simulink model "PV_MPPT_DesktopSim"  (R2023b)
settings: Solver=ode23tb  StartTime=0.0  StopTime=inf  MaxStep=1e-4  RelTol=1e-3
PreLoadFcn:
  | load('EmulatedPV_LowPowerData.mat');
  | 
  | numIrr = 10;
  | ArrayPower = ArrayCurrent.*ArrayVoltage;
InitFcn:
  | Ts = 1e-4;
  | Tc = Ts;
undefined symbols (not defined in the file): ArrayCurrent, ArrayVoltage, DiscIntNeverNeededParam, Irradiance, Tdata
libraries: spsSeriesRLCBranchLib x27, fl_lib x15, spsMosfetLib x11, ee_lib x11, spsVoltageMeasurementLib x7, spsCurrentMeasurementLib x6, nesl_utility x5, spsDiodeLib x5, spspowerguiLib x4, spsTriangleGeneratorLib x3, spsParallelRLCBranchLib x3, spsGroundLib x2
(part 1 of 3)
settings Model: Creator=mmishra  LastModifiedBy=32295
settings SolverCC: AlgebraicLoopSolver=TrustRegion
settings DataIOCC: ReturnWorkspaceOutputs=off
settings DebuggingCC: UnconnectedInputMsg=warning  UnconnectedOutputMsg=warning  UnconnectedLineMsg=warning  ArithmeticOperatorsInVariantConditions=warning
settings ModelReferenceCC: EnableRefExpFcnMdlSchedulingChecks=on
settings SFSimCC: SimUseLocalCustomCode=off  CustomCodeUndefinedFunction=UseInterfaceOnly
settings RTWCC: RTWUseLocalCustomCode=off

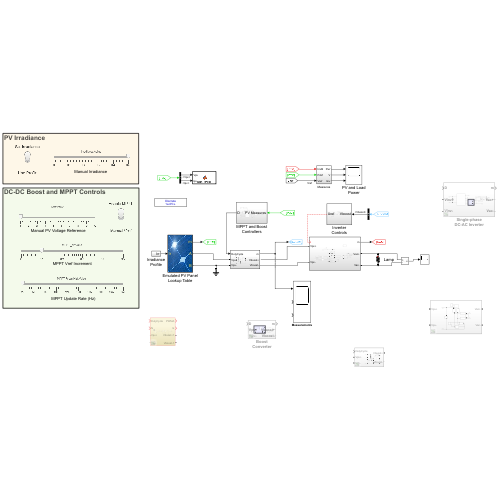
[thumbnail: Simulink's stored preview of the top-level diagram]
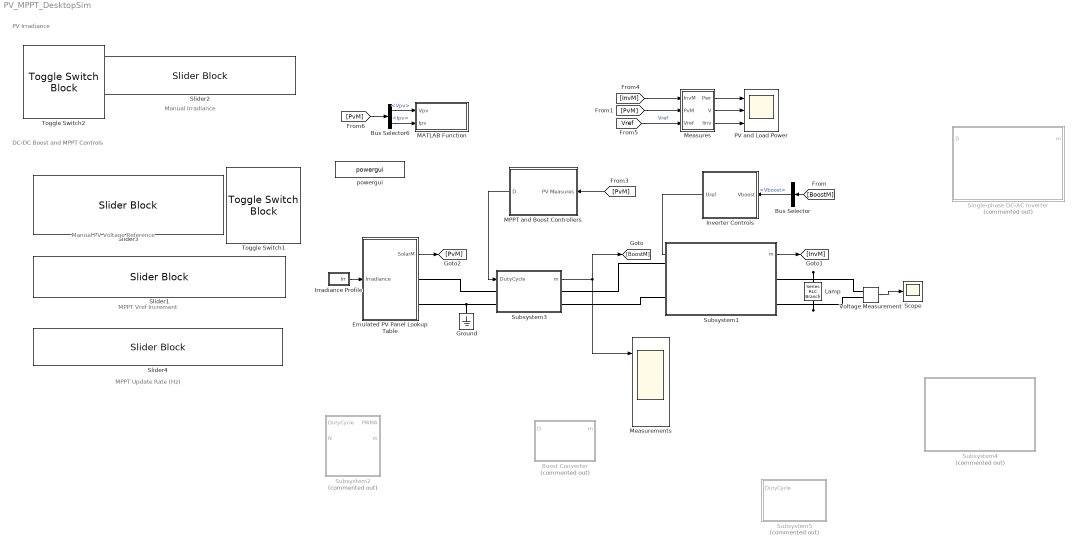
== system PV_MPPT_DesktopSim ==
  note: Manual Irradiance
  note: PV Irradiance
  note: MPPT Update Rate (Hz)
  note: MPPT Vref Increment
  note: DC-DC Boost and MPPT Controls
  note: Manual PV Voltage Reference
  Boost Converter : Subsystem  Commented=on
  Bus Selector : BusSelector  OutputSignals=Vboost
  Bus Selector6 : BusSelector  OutputSignals=Vpv,Ipv
  Emulated PV Panel Lookup Table : Subsystem
      mask Display:
      | image(imread('panel.jpg'))
      | color('yellow')
      | port_label('input',1,'Ir')
      | port_label('output',1,'m')
      | port_label('Rconn',1,'A')
      | port_label('Rconn',2,'B')
  Ground : spsGroundLib/Ground  LConnTagsString=a
  Inverter Controls : Subsystem
  Irradiance Profile : Subsystem
  Lamp : spsSeriesRLCBranchLib/Series RLC Branch  LConnTagsString=__new0  RConnTagsString=__new0  BranchType=R  Resistance=11.5  Inductance=1e-3  SetiL0=off  InitialCurrent=0  Capacitance=1e-6  Setx0=off  InitialVoltage=0  Measurements=None
  MATLAB Function : MATLAB Function  TreatAsAtomicUnit=on  SystemSampleTime=1/20
  MPPT and Boost Controllers : Subsystem
  Measurements : Scope  NumInputPorts=3
  Measures : Subsystem
  PV and Load Power : Scope  NumInputPorts=3
  Scope : Scope
  Single-phase DC-AC Inverter : Subsystem  Commented=on
  Slider1 : SliderBlock  ScaleMax=0.5  TickInterval=0.10000000000000001
  Slider2 : SliderBlock  ScaleMax=0.5  TickInterval=0.10000000000000001
  Slider3 : SliderBlock  ScaleMin=1  ScaleMax=10  TickInterval=1
  Slider4 : SliderBlock  ScaleMin=25  ScaleMax=250  TickInterval=25
  Subsystem1 : Subsystem
  Subsystem2 : Subsystem  Commented=on
  Subsystem3 : Subsystem
  Subsystem4 : Subsystem  Commented=on
  Subsystem5 : Subsystem  Commented=on
  Toggle Switch1 : ToggleSwitchBlock  LabelPosition=Hide
      settings: Values={{'Manual Vref', 'Enable MPPT'}, [0 1]}
  Toggle Switch2 : ToggleSwitchBlock  LabelPosition=Hide
      settings: Values={{'Use Profile', 'Set Irradiance'}, [0 1]}
  Voltage Measurement : spsVoltageMeasurementLib/Voltage Measurement  PhasorSimulation=off  OutputType=Complex  PSBequivalent=0
  powergui : spspowerguiLib/powergui  Priority=1  SimulationMode=Discrete  SampleTime=1e-5  frequency=60  Iterations=50  frequencyindice=0  Pbase=100e6  ErrMax=1e-4  UnitsV=kV  UnitsW=MW  buscounter=0  FunctionMessages=off  echomessages=off  EnableUseOfTLC=off  CurrentSourceSwitches=off  DisableSnubberDevices=off  DisableRonSwitches=off  DisableVfSwitches=off  DisplayEquations=off  AutomaticDiscreteSolvers=off  SolverType=Tustin  Interpol=off  ExternalGateDelay=off  methode=off  Ts=0  x0status=blocks  SPID=off  SwTol=0  HookPort=off  NonlinearTolerance=1e-4  nMaxIteration=100  ContinueOnMaxIteration=off  RestoreLinks=warning  ResistiveCurrentMeasurement=off  Frange=[0:2:500]  Ylog=off  Xlog=on  ShowGrid=off  save=off  variable=ZData  structure=0  ZoomFFT=on  StartTime=0.0  cycles=1  DisplayStyle=1  fundamental=60  FreqAxis=off  MaxFrequency=1000  frequencyindicesteady=1  RmsSteady=1  display=off
  wires:
  Irradiance Profile/1(Irr) -> Emulated PV Panel Lookup Table/1(Irradiance)
  Subsystem1/1(m) -> [InvM]
  Emulated PV Panel Lookup Table/1(SolarM) -> [PvM]
  MPPT and Boost Controllers/1(D) -> Subsystem3/1(DutyCycle)
  Subsystem3/1(m) -> Measurements/1, [BoostM]
  [PvM] -> MPPT and Boost Controllers/1(PV Measures)
  Bus Selector/1 -> Inverter Controls/1(Vboost)  "<Vboost>"
  Inverter Controls/1(Uref) -> ?
  [BoostM] -> Bus Selector/1
  Bus Selector6/1 -> MATLAB Function/1(Vpv)  "<Vpv>"
  Bus Selector6/2 -> MATLAB Function/2(Ipv)  "<Ipv>"
  [PvM] -> Bus Selector6/1
  [InvM] -> Measures/1(InvM)
  [PvM] -> Measures/2(PvM)
  [Vref] -> Measures/3(Vref)  "Vref"
  Measures/1(Pwr) -> PV and Load Power/1
  Measures/2(V) -> PV and Load Power/2
  Measures/3(Iinv) -> PV and Load Power/3
  Voltage Measurement/1 -> Scope/1
  connections:
  Ground/LConn1 -- Subsystem3/LConn2 -- Emulated PV Panel Lookup Table/RConn2
  Subsystem3/LConn1 -- Emulated PV Panel Lookup Table/RConn1
  Lamp/RConn1 -- Subsystem1/RConn2 -- Voltage Measurement/LConn2
  Subsystem3/RConn1 -- Subsystem1/LConn1
  Subsystem3/RConn2 -- Subsystem1/LConn2
  Lamp/LConn1 -- Subsystem1/RConn1 -- Voltage Measurement/LConn1

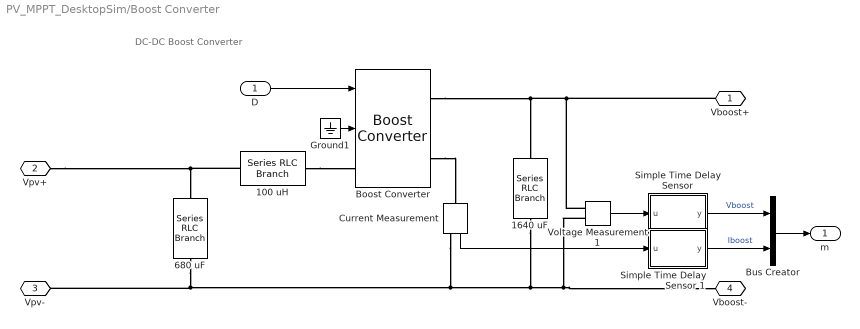
== system PV_MPPT_DesktopSim/Boost Converter ==
  note: DC-DC Boost Converter
  D : Inport
  100 uH : spsSeriesRLCBranchLib/Series RLC Branch  LConnTagsString=__new0  RConnTagsString=__new0  BranchType=L  Resistance=1  Inductance=100e-6  SetiL0=off  InitialCurrent=0  Capacitance=1e-6  Setx0=off  InitialVoltage=0  Measurements=None
  1640 uF : spsSeriesRLCBranchLib/Series RLC Branch  LConnTagsString=__new0  RConnTagsString=__new0  BranchType=C  Resistance=1  Inductance=1e-3  SetiL0=off  InitialCurrent=0  Capacitance=1640e-6  Setx0=off  InitialVoltage=30  Measurements=None
  680 uF : spsSeriesRLCBranchLib/Series RLC Branch  LConnTagsString=__new0  RConnTagsString=__new0  BranchType=C  Resistance=1e-3  Inductance=1e-3  SetiL0=off  InitialCurrent=0  Capacitance=680e-6  Setx0=off  InitialVoltage=20  Measurements=None
  "Boost Converter " : spsBoostConverterLib/Boost Converter  ModelType=Average model (D-controlled)  Ron=1e-3  Rs=1e6  Cs=inf  Vforward=[0,0.8]  Ron_Diode=1e-3  Rs_Diode=1e6  Cs_Diode=inf  Vf_Diode=0.8  Rs_CurrentSource=inf  Ron_ACsource=1e-3
      settings: LibrarySourceBlock=sps_lib/Power Electronics/Boost Converter
  Bus Creator : BusCreator  Inputs=2
  Current Measurement : spsCurrentMeasurementLib/Current Measurement  PhasorSimulation=off  OutputType=Complex  PSBequivalent=0
  Ground1 : Ground
  "Simple Time Delay Sensor " : Subsystem  mask{Ts=Ts, Tau=0.0001}
      mask prompts: Ts "Sample Time, [s]"; Tau "Time Constant, Tau [s]"
      mask help: Simple Sensor
      mask Display: fprintf('1\n------------\n(1 + s Tau)');
  Simple Time Delay Sensor 1 : Subsystem  mask{Ts=Ts, Tau=0.0001}
      mask prompts: Ts "Sample Time, [s]"; Tau "Time Constant, Tau [s]"
      mask help: Simple Sensor
      mask Display: fprintf('1\n------------\n(1 + s Tau)');
  Voltage Measurement1 : spsVoltageMeasurementLib/Voltage Measurement  PhasorSimulation=off  OutputType=Complex  PSBequivalent=0
  Vboost+ : PMIOPort  Side=Right
  Vpv+ : PMIOPort  Port=2  Side=Left
  Vpv- : PMIOPort  Port=3  Side=Left
  Vboost- : PMIOPort  Port=4  Side=Right
  m : Outport  VectorParamsAs1DForOutWhenUnconnected=off
  wires:
  Ground1/1 -> "Boost Converter "/2
  Current Measurement/1 -> Simple Time Delay Sensor 1/1(u)
  Voltage Measurement1/1 -> "Simple Time Delay Sensor "/1(u)
  Bus Creator/1 -> m/1
  "Simple Time Delay Sensor "/1(y) -> Bus Creator/1  "Vboost"
  Simple Time Delay Sensor 1/1(y) -> Bus Creator/2  "Iboost"
  D/1 -> "Boost Converter "/1
  connections:
  100 uH/LConn1 -- Vpv+/RConn1 -- 680 uF/LConn1
  "Boost Converter "/RConn2 -- Current Measurement/LConn1
  100 uH/RConn1 -- "Boost Converter "/LConn1
  Voltage Measurement1/LConn1 -- Vboost+/RConn1 -- "Boost Converter "/RConn1 -- 1640 uF/LConn1
  680 uF/RConn1 -- Vboost-/RConn1 -- Voltage Measurement1/LConn2 -- 1640 uF/RConn1 -- Current Measurement/RConn1 -- Vpv-/RConn1

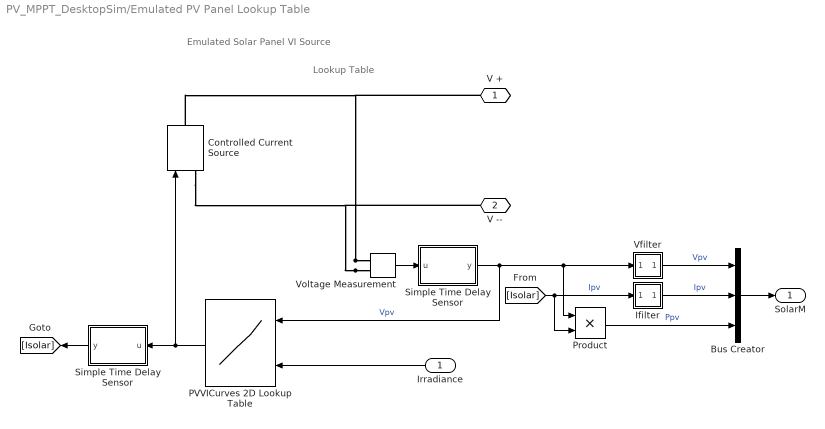
== system PV_MPPT_DesktopSim/Emulated PV Panel Lookup Table ==
  note: Lookup Table
  note: Emulated Solar Panel VI Source
  Irradiance : Inport
  Bus Creator : BusCreator  Inputs=3
  Controlled Current Source : spsControlledCurrentSourceLib/Controlled Current Source  Initialize=on  Source_Type=AC  Amplitude=0  Phase=0  Frequency=0  Measurements=None
  Ifilter : Subsystem  mask{Tf=0.01}
      mask prompts: Tf "Filter Time Constant"
  PVVICurves 2D Lookup Table : Lookup_n-D  BreakpointsForDimension1=ArrayVoltage  BreakpointsForDimension2=Irradiance  Table=ArrayCurrent  InternalRulePriority=Speed  RndMeth=Simplest
      settings: InputPortMap=u0,u1
  Product : Product
  Simple Time Delay Sensor : Subsystem  mask{Ts=Ts, Tau=0.0001}
      mask prompts: Ts "Sample Time, [s]"; Tau "Time Constant, Tau [s]"
      mask help: Simple Sensor
      mask Display: fprintf('1\n------------\n(1 + s Tau)');
  "Simple Time Delay Sensor " : Subsystem  mask{Ts=Ts, Tau=0.0001}
      mask prompts: Ts "Sample Time, [s]"; Tau "Time Constant, Tau [s]"
      mask help: Simple Sensor
      mask Display: fprintf('1\n------------\n(1 + s Tau)');
  Vfilter : Subsystem  mask{Tf=0.01}
      mask prompts: Tf "Filter Time Constant"
  Voltage Measurement : spsVoltageMeasurementLib/Voltage Measurement  PhasorSimulation=off  OutputType=Complex  PSBequivalent=0
  V + : PMIOPort  Side=Right
  V -- : PMIOPort  Port=2  Side=Right
  SolarM : Outport  VectorParamsAs1DForOutWhenUnconnected=off
  wires:
  Irradiance/1 -> PVVICurves 2D Lookup Table/2
  PVVICurves 2D Lookup Table/1 -> Simple Time Delay Sensor/1(u), Controlled Current Source/1
  Bus Creator/1 -> SolarM/1
  [Isolar] -> Product/2, Ifilter/1(u)  "Ipv"
  Product/1 -> Bus Creator/3  "Ppv"
  Simple Time Delay Sensor/1(y) -> [Isolar]
  "Simple Time Delay Sensor "/1(y) -> Product/1, Vfilter/1(u), PVVICurves 2D Lookup Table/1  "Vpv"
  Voltage Measurement/1 -> "Simple Time Delay Sensor "/1(u)
  Vfilter/1(y) -> Bus Creator/1  "Vpv"
  Ifilter/1(y) -> Bus Creator/2  "Ipv"
  connections:
  Voltage Measurement/LConn2 -- Controlled Current Source/LConn1 -- V --/RConn1
  Voltage Measurement/LConn1 -- Controlled Current Source/RConn1 -- V +/RConn1

== system PV_MPPT_DesktopSim/Inverter Controls ==
  Vboost : Inport
  Boost Voltage Controller : slpidlib/PID Controller  Controller=PI  Form=Parallel  TimeDomain=Discrete-time  UseExternalTs=off  SampleTime=Tc  IntegratorMethod=Forward Euler  FilterMethod=Forward Euler  ControllerParametersSource=internal  P=3  I=250  UseKiTs=off  D=0  N=100  UseFilter=on  TunerSelectOption=Transfer Function Based (PID Tuner App)  InitialConditionSource=internal  InitialConditionForIntegrator=1  InitialConditionForFilter=0  DifferentiatorICPrevScaledInput=0  ExternalReset=none  TrackingMode=off  Kt=1  LimitOutput=on  SatLimitsSource=internal  UpperSaturationLimit=1  LowerSaturationLimit=0  LinearizeAsGain=on  AntiWindupMode=clamping  Kb=1  LimitIntegrator=off  UpperIntegratorSaturationLimit=inf  LowerIntegratorSaturationLimit=-inf  POutMin=[]  POutMax=[]  IOutMin=[]  IOutMax=[]  DOutMin=[]  DOutMax=[]  NOutMin=[]  NOutMax=[]  SumOutMin=[]  SumOutMax=[]  SaturationOutMin=[]  SaturationOutMax=[]  PParamMin=[]  PParamMax=[]  IParamMin=[]  IParamMax=[]  DParamMin=[]  DParamMax=[]  NParamMin=[]  NParamMax=[]  KbParamMin=[]  KbParamMax=[]  KtParamMin=[]  KtParamMax=[]  KbOutMin=[]  KbOutMax=[]  KtOutMin=[]  KtOutMax=[]  IntegratorOutMin=[]  IntegratorOutMax=[]  FilterOutMin=[]  FilterOutMax=[]  SumI1OutMin=[]  SumI1OutMax=[]  SumI2OutMin=[]  SumI2OutMax=[]  SumI3OutMin=[]  SumI3OutMax=[]  SumI4OutMin=[]  SumI4OutMax=[]  SumDOutMin=[]  SumDOutMax=[]  DifferentiatorOutMin=[]  DifferentiatorOutMax=[]  FilterDiffOutCoefMin=[]  FilterDiffOutCoefMax=[]  ReciprocalOutMin=[]  ReciprocalOutMax=[]  SumDenOutMin=[]  SumDenOutMax=[]  SumNumOutMin=[]  SumNumOutMax=[]  DivideOutMin=[]  DivideOutMax=[]  UdiffTsProdOutMin=[]  UdiffTsProdOutMax=[]  NTsProdOutMin=[]  NTsProdOutMax=[]  UintegralTsProdOutMin=[]  UintegralTsProdOutMax=[]  UngainTsProdOutMin=[]  UngainTsProdOutMax=[]  ClampingZeroOutDataTypeStr=Inherit: Inherit via back propagation  ClampingZeroOutMin=[]  ClampingZeroOutMax=[]  FilterDenConstantOutDataTypeStr=Inherit: Inherit via back propagation  FilterDenConstantOutMin=[]  FilterDenConstantOutMax=[]  PCopyOutDataTypeStr=Inherit: Inherit via back propagation  PCopyOutMin=[]  PCopyOutMax=[]  NCopyOutDataTypeStr=Inherit: Inherit via back propagation  NCopyOutMin=[]  NCopyOutMax=[]  IntegratorContinuousStateAttributes=''  IntegratorStateMustResolveToSignalObject=off  IntegratorRTWStateStorageClass=Auto  FilterContinuousStateAttributes=''  FilterStateMustResolveToSignalObject=off  FilterRTWStateStorageClass=Auto  ParallelPVariant=InternalParameters  IdealPVariant=Disabled  IVariant=InternalParameters  DVariant=Disabled  IntegratorVariant=Discrete  SatVariant=Enabled  AWVariant=DiscClampingParallel  PCopyVariant=Disabled  TRVariant=Disabled  FdbkBlocksVariant=Forward  IdealPFdbkVariant=Disabled  SatFdbkVariant=Disabled  DerivativeFilterVariant=Disabled  NVariant=Disabled  NCopyVariant=Disabled_SignalSpec  FilterICVariant=Disabled  IntegratorICVariant=InternalICs  ExternalResetVariant=Disabled  TRSumVariant=Passthrough  SumFdbkVariant=Disabled  SumVariant=Sum_PI  TsampFilterVariant=InternalTs  TsampNgainVariant=Passthrough  TsampIntegralVariant=Disabled_SignalSpec  ExternalSaturationOutDataTypeStr=Inherit: Same as second input
  Constant1 : Constant  Value=30
  Gain : Gain  Gain=1/30
  "PWM Generator (2-Level) " : spsPWMGenerator2LevelLib/PWM Generator (2-Level)  Commented=through  ModulatorType=Single-phase full-bridge (4 pulses)  ModulatorMode=Unsynchronized  Fc=6000  Pc=90  nF=27  MinMax="[ -1  1 ]"  SamplingTechnique=Natural  ModulatingSignals=off  m=0.8  Freq=60  Phase=0  Ts=Ts  ShowCarrierOutport=off
  Product : Product
  Sine Wave : Sin  Frequency=2*pi*60  SampleTime=Tc
  Sum3 : Sum  Inputs=|+-
  Uref : Outport  VectorParamsAs1DForOutWhenUnconnected=off
  wires:
  Constant1/1 -> Sum3/2
  Sine Wave/1 -> Product/1
  Boost Voltage Controller/1 -> Product/2
  Sum3/1 -> Gain/1
  Vboost/1 -> Sum3/1
  Gain/1 -> Boost Voltage Controller/1
  Product/1 -> "PWM Generator (2-Level) "/1
  "PWM Generator (2-Level) "/1 -> Uref/1

== system PV_MPPT_DesktopSim/Irradiance Profile ==
  note: PV Irradiance
  Irradiance : Constant  Value=0.5  OutDataTypeStr=single
  Irradiance_Select : Constant  OutDataTypeStr=single
  NewIrradiance1 : Constant  Value=0.15  OutDataTypeStr=single
  Pulse Generator : DiscretePulseGenerator  PulseType=Time based  Amplitude=0.15  Period=10  PulseWidth=50
  Sum : Sum  Inputs=|++
  Switch : Switch  Criteria=u2 > Threshold  SaturateOnIntegerOverflow=off  InputSameDT=off
  Irr : Outport  VectorParamsAs1DForOutWhenUnconnected=off
  wires:
  NewIrradiance1/1 -> Sum/2
  Pulse Generator/1 -> Sum/1
  Sum/1 -> Switch/3
  Irradiance/1 -> Switch/1
  Switch/1 -> Irr/1
  Irradiance_Select/1 -> Switch/2

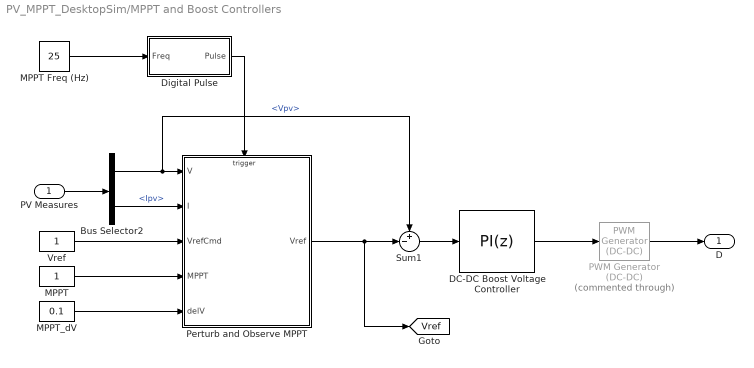
== system PV_MPPT_DesktopSim/MPPT and Boost Controllers ==
  PV Measures : Inport
  Bus Selector2 : BusSelector  OutputSignals=Vpv,Ipv
  DC-DC Boost Voltage Controller : slpidlib/PID Controller  Controller=PI  Form=Parallel  TimeDomain=Discrete-time  UseExternalTs=off  SampleTime=Tc  IntegratorMethod=Forward Euler  FilterMethod=Forward Euler  ControllerParametersSource=internal  P=0.015  I=2.5  UseKiTs=off  D=0  N=100  UseFilter=on  TunerSelectOption=Transfer Function Based (PID Tuner App)  InitialConditionSource=internal  InitialConditionForIntegrator=0  InitialConditionForFilter=0  DifferentiatorICPrevScaledInput=0  ExternalReset=none  TrackingMode=off  Kt=1  LimitOutput=off  SatLimitsSource=internal  UpperSaturationLimit=0.9  LowerSaturationLimit=0  LinearizeAsGain=on  AntiWindupMode=clamping  Kb=1  LimitIntegrator=off  UpperIntegratorSaturationLimit=inf  LowerIntegratorSaturationLimit=-inf  POutMin=[]  POutMax=[]  IOutMin=[]  IOutMax=[]  DOutMin=[]  DOutMax=[]  NOutMin=[]  NOutMax=[]  SumOutMin=[]  SumOutMax=[]  SaturationOutMin=[]  SaturationOutMax=[]  PParamMin=[]  PParamMax=[]  IParamMin=[]  IParamMax=[]  DParamMin=[]  DParamMax=[]  NParamMin=[]  NParamMax=[]  KbParamMin=[]  KbParamMax=[]  KtParamMin=[]  KtParamMax=[]  KbOutMin=[]  KbOutMax=[]  KtOutMin=[]  KtOutMax=[]  IntegratorOutMin=[]  IntegratorOutMax=[]  FilterOutMin=[]  FilterOutMax=[]  SumI1OutMin=[]  SumI1OutMax=[]  SumI2OutMin=[]  SumI2OutMax=[]  SumI3OutMin=[]  SumI3OutMax=[]  SumI4OutMin=[]  SumI4OutMax=[]  SumDOutMin=[]  SumDOutMax=[]  DifferentiatorOutMin=[]  DifferentiatorOutMax=[]  FilterDiffOutCoefMin=[]  FilterDiffOutCoefMax=[]  ReciprocalOutMin=[]  ReciprocalOutMax=[]  SumDenOutMin=[]  SumDenOutMax=[]  SumNumOutMin=[]  SumNumOutMax=[]  DivideOutMin=[]  DivideOutMax=[]  UdiffTsProdOutMin=[]  UdiffTsProdOutMax=[]  NTsProdOutMin=[]  NTsProdOutMax=[]  UintegralTsProdOutMin=[]  UintegralTsProdOutMax=[]  UngainTsProdOutMin=[]  UngainTsProdOutMax=[]  ClampingZeroOutDataTypeStr=Inherit: Inherit via back propagation  ClampingZeroOutMin=[]  ClampingZeroOutMax=[]  FilterDenConstantOutDataTypeStr=Inherit: Inherit via back propagation  FilterDenConstantOutMin=[]  FilterDenConstantOutMax=[]  PCopyOutDataTypeStr=Inherit: Inherit via back propagation  PCopyOutMin=[]  PCopyOutMax=[]  NCopyOutDataTypeStr=Inherit: Inherit via back propagation  NCopyOutMin=[]  NCopyOutMax=[]  IntegratorContinuousStateAttributes=''  IntegratorStateMustResolveToSignalObject=off  IntegratorRTWStateStorageClass=Auto  FilterContinuousStateAttributes=''  FilterStateMustResolveToSignalObject=off  FilterRTWStateStorageClass=Auto  ParallelPVariant=InternalParameters  IdealPVariant=Disabled  IVariant=InternalParameters  DVariant=Disabled  IntegratorVariant=Discrete  SatVariant=Disabled  AWVariant=Passthrough  PCopyVariant=Disabled  TRVariant=Disabled  FdbkBlocksVariant=Forward  IdealPFdbkVariant=Disabled  SatFdbkVariant=Disabled  DerivativeFilterVariant=Disabled  NVariant=Disabled  NCopyVariant=Disabled_SignalSpec  FilterICVariant=Disabled  IntegratorICVariant=InternalICs  ExternalResetVariant=Disabled  TRSumVariant=Passthrough  SumFdbkVariant=Disabled  SumVariant=Sum_PI  TsampFilterVariant=InternalTs  TsampNgainVariant=Passthrough  TsampIntegralVariant=Disabled_SignalSpec  ExternalSaturationOutDataTypeStr=Inherit: Same as second input
  Digital Pulse : Subsystem  mask{Ts=Tc, Duty=0.5}
      mask prompts: Ts "Sample Rate [s]"; Duty "Duty Cycle [0-1]"
  MPPT : Constant
  MPPT Freq (Hz) : Constant  Value=25
  MPPT_dV : Constant  Value=0.1
  PWM Generator (DC-DC) : spsPWMGeneratorDCDCLib/PWM Generator (DC-DC)  Commented=through  Fsw=5000  Ts=Ts
  Perturb and Observe MPPT : Stateflow chart  TreatAsAtomicUnit=on  SystemSampleTime=Tdata
  Sum1 : Sum  Inputs=+-|
  Vref : Constant
  D : Outport  VectorParamsAs1DForOutWhenUnconnected=off
  tag scope: Vref=global
  wires:
  PV Measures/1 -> Bus Selector2/1
  Digital Pulse/1(Pulse) -> Perturb and Observe MPPT/Trigger
  MPPT Freq (Hz)/1 -> Digital Pulse/1(Freq)
  MPPT_dV/1 -> Perturb and Observe MPPT/5(delV)
  Vref/1 -> Perturb and Observe MPPT/3(VrefCmd)
  Sum1/1 -> DC-DC Boost Voltage Controller/1
  MPPT/1 -> Perturb and Observe MPPT/4(MPPT)
  Bus Selector2/1 -> Perturb and Observe MPPT/1(V), Sum1/1  "<Vpv>"
  Perturb and Observe MPPT/1(Vref) -> [Vref], Sum1/2
  Bus Selector2/2 -> Perturb and Observe MPPT/2(I)  "<Ipv>"
  DC-DC Boost Voltage Controller/1 -> PWM Generator (DC-DC)/1
  PWM Generator (DC-DC)/1 -> D/1

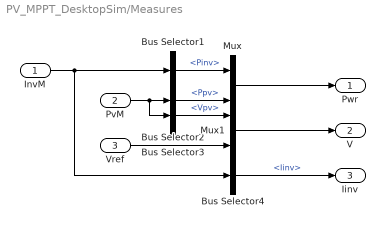
== system PV_MPPT_DesktopSim/Measures ==
  InvM : Inport
  PvM : Inport  Port=2
  Vref : Inport  Port=3
  Bus Selector1 : BusSelector  OutputSignals=Pinv
  Bus Selector2 : BusSelector  OutputSignals=Ppv
  Bus Selector3 : BusSelector  OutputSignals=Vpv
  Bus Selector4 : BusSelector  OutputSignals=Iinv
  Mux : Mux  Inputs=2
  Mux1 : Mux  Inputs=2
  Pwr : Outport  VectorParamsAs1DForOutWhenUnconnected=off
  V : Outport  Port=2  VectorParamsAs1DForOutWhenUnconnected=off
  Iinv : Outport  Port=3  VectorParamsAs1DForOutWhenUnconnected=off
  wires:
  Bus Selector2/1 -> Mux/2  "<Ppv>"
  PvM/1 -> Bus Selector3/1, Bus Selector2/1
  Mux/1 -> Pwr/1
  Bus Selector1/1 -> Mux/1  "<Pinv>"
  Bus Selector3/1 -> Mux1/1  "<Vpv>"
  Bus Selector4/1 -> Iinv/1  "<Iinv>"
  Mux1/1 -> V/1
  Vref/1 -> Mux1/2
  InvM/1 -> Bus Selector4/1, Bus Selector1/1

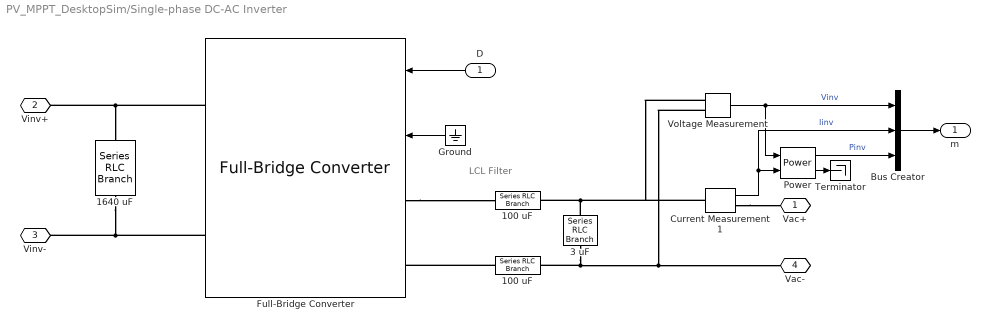
== system PV_MPPT_DesktopSim/Single-phase DC-AC Inverter ==
  note: LCL Filter
  D : Inport
  100 uF : spsSeriesRLCBranchLib/Series RLC Branch  LConnTagsString=__new0  RConnTagsString=__new0  BranchType=L  Resistance=1  Inductance=100e-6  SetiL0=off  InitialCurrent=0  Capacitance=1e-6  Setx0=off  InitialVoltage=0  Measurements=None
  "100 uF " : spsSeriesRLCBranchLib/Series RLC Branch  LConnTagsString=__new0  RConnTagsString=__new0  BranchType=L  Resistance=1  Inductance=100e-6  SetiL0=off  InitialCurrent=0  Capacitance=1e-6  Setx0=off  InitialVoltage=0  Measurements=None
  "1640 uF " : spsSeriesRLCBranchLib/Series RLC Branch  LConnTagsString=__new0  RConnTagsString=__new0  BranchType=RC  Resistance=0.05  Inductance=1e-3  SetiL0=off  InitialCurrent=0  Capacitance=1640e-6  Setx0=off  InitialVoltage=0  Measurements=None
  3 uF : spsSeriesRLCBranchLib/Series RLC Branch  LConnTagsString=__new0  RConnTagsString=__new0  BranchType=C  Resistance=1  Inductance=1e-3  SetiL0=off  InitialCurrent=0  Capacitance=3e-6  Setx0=off  InitialVoltage=0  Measurements=None
  Bus Creator : BusCreator  Inputs=3
  Current Measurement1 : spsCurrentMeasurementLib/Current Measurement  PhasorSimulation=off  OutputType=Complex  PSBequivalent=0
  Full-Bridge Converter : spsFullBridgeConverterLib/Full-Bridge Converter  ModelType=Average model (Uref-controlled)  Ron=1e-3  Rs=1e6  Cs=inf  Vforward=[0,0]  Ron_Diode=1e-3  Rs_Diode=1e6  Cs_Diode=inf  Vf_Diode=1e-3  Rs_CurrentSource=inf  Ron_ACsource=1e-3
      settings: LibrarySourceBlock=sps_lib/Power Electronics/Full-Bridge Converter
  Ground : Ground
  Power : spsPowerLib/Power  Freq=60  Vinit=[1, 0]  Iinit=[1, 0]  Ts=Ts
  Terminator : Terminator
  Voltage Measurement : spsVoltageMeasurementLib/Voltage Measurement  PhasorSimulation=off  OutputType=Complex  PSBequivalent=0
  Vac+ : PMIOPort  Side=Right
  Vinv+ : PMIOPort  Port=2  Side=Left
  Vinv- : PMIOPort  Port=3  Side=Left
  Vac- : PMIOPort  Port=4  Side=Right
  m : Outport  VectorParamsAs1DForOutWhenUnconnected=off
  wires:
  Ground/1 -> Full-Bridge Converter/2
  D/1 -> Full-Bridge Converter/1
  Bus Creator/1 -> m/1
  Power/1 -> Bus Creator/3  "Pinv"
  Voltage Measurement/1 -> Bus Creator/1, Power/1  "Vinv"
  Current Measurement1/1 -> Power/2, Bus Creator/2  "Iinv"
  Power/2 -> Terminator/1
  connections:
  Full-Bridge Converter/RConn1 -- "1640 uF "/LConn1 -- Vinv+/RConn1
  3 uF/RConn1 -- Vac-/RConn1 -- Voltage Measurement/LConn2 -- "100 uF "/RConn1
  "1640 uF "/RConn1 -- Full-Bridge Converter/RConn2 -- Vinv-/RConn1
  "100 uF "/LConn1 -- Full-Bridge Converter/LConn2
  Full-Bridge Converter/LConn1 -- 100 uF/LConn1
  3 uF/LConn1 -- Current Measurement1/LConn1 -- Voltage Measurement/LConn1 -- 100 uF/RConn1
  Current Measurement1/RConn1 -- Vac+/RConn1

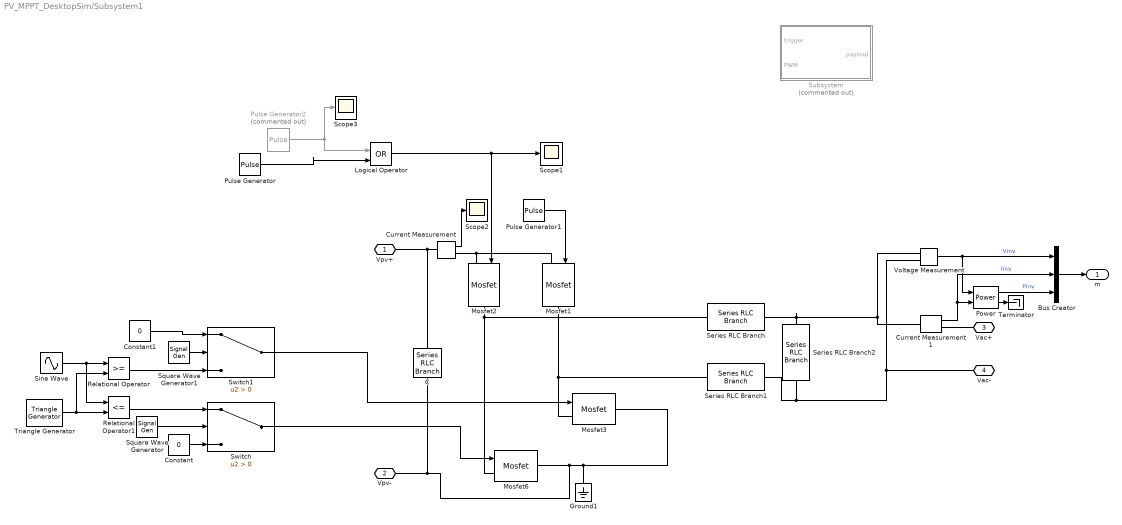
== system PV_MPPT_DesktopSim/Subsystem1 ==
  Bus Creator : BusCreator  Inputs=3
  C : spsSeriesRLCBranchLib/Series RLC Branch  LConnTagsString=__new0  RConnTagsString=__new0  BranchType=C  Resistance=1e-4  Inductance=200e-6  SetiL0=off  InitialCurrent=0  Capacitance=200e-6  Setx0=off  InitialVoltage=0  Measurements=None
  Constant : Constant  Value=0
  Constant1 : Constant  Value=0
  Current Measurement : spsCurrentMeasurementLib/Current Measurement  PhasorSimulation=off  OutputType=Complex  PSBequivalent=0
  Current Measurement1 : spsCurrentMeasurementLib/Current Measurement  PhasorSimulation=off  OutputType=Complex  PSBequivalent=0
  Ground1 : spsGroundLib/Ground  LConnTagsString=a
  Logical Operator : Logic  Operator=OR  IconShape=distinctive  AllPortsSameDT=off  OutDataTypeStr=boolean
  Mosfet{1..3,6} (4 alike) : spsMosfetLib/Mosfet  Ron=0.1  Lon=0  Rd=0.01  Vfd=0  IC=0  Rs=1e5  Cs=inf  Measurements=off
  Power : spsPowerLib/Power  Freq=60  Vinit=[1, 0]  Iinit=[1, 0]  Ts=Ts
  Pulse Generator : DiscretePulseGenerator  PulseType=Time based  Amplitude=5  Period=0.02  PulseWidth=50
  Pulse Generator1 : DiscretePulseGenerator  PulseType=Time based  Amplitude=5  Period=0.02  PulseWidth=50  PhaseDelay=0.01
  Pulse Generator2 : DiscretePulseGenerator  Commented=on  PulseType=Time based  Amplitude=5  Period=0.8  PulseWidth=50  PhaseDelay=0.4
  Relational Operator : RelationalOperator  OutDataTypeStr=boolean  RndMeth=Simplest  InputSameDT=off
  Relational Operator1 : RelationalOperator  Operator=<=  OutDataTypeStr=boolean  RndMeth=Simplest  InputSameDT=off
  Scope1 : Scope
  Scope2 : Scope
  Scope3 : Scope
  Series RLC Branch : spsSeriesRLCBranchLib/Series RLC Branch  LConnTagsString=__new0  RConnTagsString=__new0  BranchType=L  Resistance=1  Inductance=7e-3  SetiL0=off  InitialCurrent=0  Capacitance=1e-6  Setx0=off  InitialVoltage=0  Measurements=None
  Series RLC Branch1 : spsSeriesRLCBranchLib/Series RLC Branch  LConnTagsString=__new0  RConnTagsString=__new0  BranchType=L  Resistance=1  Inductance=7e-3  SetiL0=off  InitialCurrent=0  Capacitance=1e-6  Setx0=off  InitialVoltage=0  Measurements=None
  Series RLC Branch2 : spsSeriesRLCBranchLib/Series RLC Branch  LConnTagsString=__new0  RConnTagsString=__new0  BranchType=C  Resistance=1  Inductance=100e-6  SetiL0=off  InitialCurrent=0  Capacitance=500e-6  Setx0=off  InitialVoltage=0  Measurements=None
  Sine Wave : Sin  Frequency=2*pi*50  SampleTime=1e-6
  Square Wave Generator : SignalGenerator  WaveForm=square  Frequency=50
  Square Wave Generator1 : SignalGenerator  WaveForm=square  Frequency=50
  Subsystem : Subsystem  Commented=on
  Switch : Switch  Criteria=u2 > Threshold  SaturateOnIntegerOverflow=off  InputSameDT=off
  Switch1 : Switch  Criteria=u2 > Threshold  SaturateOnIntegerOverflow=off  InputSameDT=off
  Terminator : Terminator
  Triangle Generator : spsTriangleGeneratorLib/Triangle Generator  Freq=5000  Phase=90  Ts=0
  Voltage Measurement : spsVoltageMeasurementLib/Voltage Measurement  PhasorSimulation=off  OutputType=Complex  PSBequivalent=0
  Vpv+ : PMIOPort  Side=Left
  Vpv- : PMIOPort  Port=2  Side=Left
  Vac+ : PMIOPort  Port=3  Side=Right
  Vac- : PMIOPort  Port=4  Side=Right
  m : Outport  VectorParamsAs1DForOutWhenUnconnected=off
  wires:
  Triangle Generator/1 -> Relational Operator/2, Relational Operator1/2
  Constant/1 -> Switch/3
  Relational Operator/1 -> Switch1/3
  Switch/1 -> Mosfet6/1
  Constant1/1 -> Switch1/1
  Square Wave Generator1/1 -> Switch1/2
  Sine Wave/1 -> Relational Operator/1, Relational Operator1/1
  Switch1/1 -> Mosfet3/1
  Square Wave Generator/1 -> Switch/2
  Relational Operator1/1 -> Switch/1
  Pulse Generator1/1 -> Mosfet1/1
  Pulse Generator2/1 -> Logical Operator/1, Scope3/1
  Pulse Generator/1 -> Logical Operator/2
  Logical Operator/1 -> Scope1/1, Mosfet2/1
  Current Measurement/1 -> Scope2/1
  Power/2 -> Terminator/1
  Power/1 -> Bus Creator/3  "Pinv"
  Bus Creator/1 -> m/1
  Voltage Measurement/1 -> Bus Creator/1, Power/1  "Vinv"
  Current Measurement1/1 -> Power/2, Bus Creator/2  "Iinv"
  connections:
  Mosfet1/RConn1 -- Series RLC Branch1/LConn1 -- Mosfet3/LConn1
  Series RLC Branch1/RConn1 -- Series RLC Branch2/RConn1 -- Vac-/RConn1 -- Voltage Measurement/LConn2
  Mosfet1/LConn1 -- Current Measurement/RConn1 -- Mosfet2/LConn1
  Series RLC Branch/RConn1 -- Series RLC Branch2/LConn1 -- Current Measurement1/LConn1 -- Voltage Measurement/LConn1
  Vpv-/RConn1 -- Ground1/LConn1 -- Mosfet3/RConn1 -- Mosfet6/RConn1 -- C/RConn1
  Mosfet2/RConn1 -- Mosfet6/LConn1 -- Series RLC Branch/LConn1
  Vpv+/RConn1 -- Current Measurement/LConn1 -- C/LConn1
  Current Measurement1/RConn1 -- Vac+/RConn1

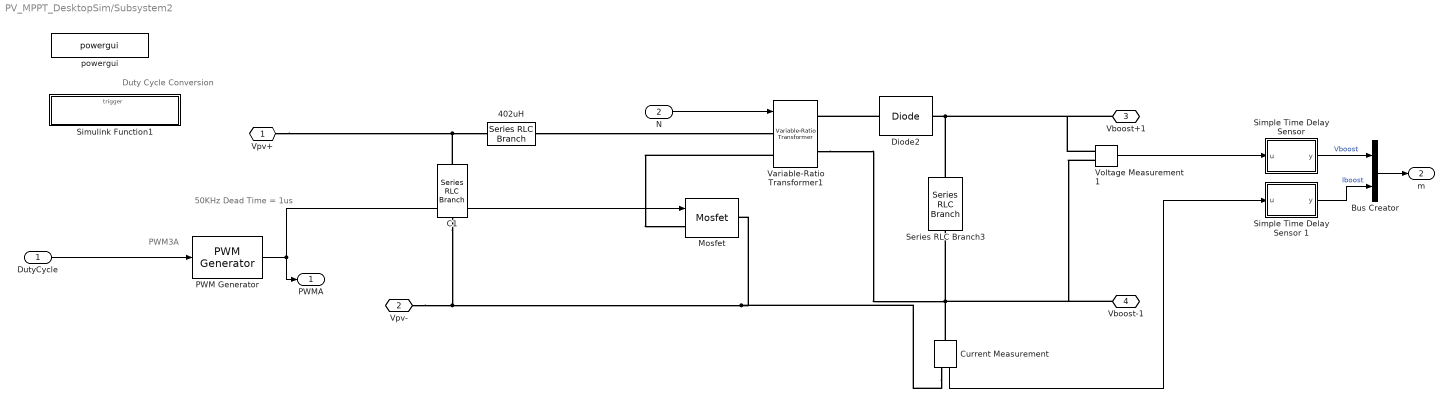
== system PV_MPPT_DesktopSim/Subsystem2 ==
  note: Duty Cycle Conversion
  note: 50KHz
      | Dead Time = 1us
  note: PWM3A
  DutyCycle : Inport
  N : Inport  Port=2
  402uH : spsSeriesRLCBranchLib/Series RLC Branch  LConnTagsString=__new0  RConnTagsString=__new0  BranchType=RL  Resistance=0.05  Inductance=100e-6  SetiL0=off  InitialCurrent=0  Capacitance=1e-6  Setx0=off  InitialVoltage=0  Measurements=None
  Bus Creator : BusCreator  Inputs=2
  C1 : spsSeriesRLCBranchLib/Series RLC Branch  LConnTagsString=__new0  RConnTagsString=__new0  BranchType=C  Resistance=1e-3  Inductance=1e-3  SetiL0=off  InitialCurrent=0  Capacitance=680e-6  Setx0=off  InitialVoltage=20  Measurements=None
  Current Measurement : spsCurrentMeasurementLib/Current Measurement  PhasorSimulation=off  OutputType=Complex  PSBequivalent=0
  Diode2 : spsDiodeLib/Diode  Ron=0.001  Lon=0  Vf=0.6  IC=0  UseSnubber=0  Rs=500  Cs=250e-9  Measurements=off
  Mosfet : spsMosfetLib/Mosfet  Ron=0.1  Lon=0  Rd=0.01  Vfd=0  IC=0  Rs=1e5  Cs=inf  Measurements=off
  PWM Generator : eePwmGenerator/PWM Generator  CarrCount=Up  Tper=20e-6  Tdelay=10e-6  Ts=1e-8
  Series RLC Branch3 : spsSeriesRLCBranchLib/Series RLC Branch  LConnTagsString=__new0  RConnTagsString=__new0  BranchType=C  Resistance=1  Inductance=1e-3  SetiL0=off  InitialCurrent=0  Capacitance=1640e-6  Setx0=off  InitialVoltage=0  Measurements=None
  "Simple Time Delay Sensor " : Subsystem  mask{Ts=Ts, Tau=0.0001}
      mask prompts: Ts "Sample Time, [s]"; Tau "Time Constant, Tau [s]"
      mask help: Simple Sensor
      mask Display: fprintf('1\n------------\n(1 + s Tau)');
  Simple Time Delay Sensor 1 : Subsystem  mask{Ts=Ts, Tau=0.0001}
      mask prompts: Ts "Sample Time, [s]"; Tau "Time Constant, Tau [s]"
      mask help: Simple Sensor
      mask Display: fprintf('1\n------------\n(1 + s Tau)');
  Simulink Function1 : Subsystem  TreatAsAtomicUnit=on
  Variable-Ratio Transformer1 : spsVariableRatioTransformerLib/Variable-Ratio Transformer
      settings: LibrarySourceBlock=|
      | sps_lib/Passives/Variable-Ratio
      | Transformer
  Voltage Measurement1 : spsVoltageMeasurementLib/Voltage Measurement  PhasorSimulation=off  OutputType=Complex  PSBequivalent=0
  powergui : spspowerguiLib/powergui  Priority=1  SimulationMode=Discrete  SampleTime=1e-5  frequency=60  Iterations=50  frequencyindice=0  Pbase=100e6  ErrMax=1e-4  UnitsV=kV  UnitsW=MW  buscounter=0  FunctionMessages=off  echomessages=off  EnableUseOfTLC=off  CurrentSourceSwitches=off  DisableSnubberDevices=off  DisableRonSwitches=off  DisableVfSwitches=off  DisplayEquations=off  AutomaticDiscreteSolvers=off  SolverType=Tustin  Interpol=off  ExternalGateDelay=off  methode=off  Ts=0  x0status=blocks  SPID=off  SwTol=0  HookPort=off  NonlinearTolerance=1e-4  nMaxIteration=100  ContinueOnMaxIteration=off  RestoreLinks=warning  ResistiveCurrentMeasurement=off  Frange=[0:2:500]  Ylog=off  Xlog=on  ShowGrid=off  save=off  variable=ZData  structure=0  ZoomFFT=on  StartTime=0.0  cycles=1  DisplayStyle=1  fundamental=60  FreqAxis=off  MaxFrequency=1000  frequencyindicesteady=1  RmsSteady=1  display=off
  Vpv+ : PMIOPort  Side=Left
  Vpv- : PMIOPort  Port=2  Side=Left
  Vboost+1 : PMIOPort  Port=3  Side=Right
  Vboost-1 : PMIOPort  Port=4  Side=Right
  PWMA : Outport  VectorParamsAs1DForOutWhenUnconnected=off
  m : Outport  Port=2  VectorParamsAs1DForOutWhenUnconnected=off
  wires:
  N/1 -> Variable-Ratio Transformer1/1
  DutyCycle/1 -> PWM Generator/1
  PWM Generator/1 -> Mosfet/1, PWMA/1
  Simple Time Delay Sensor 1/1(y) -> Bus Creator/2  "Iboost"
  Bus Creator/1 -> m/1
  "Simple Time Delay Sensor "/1(y) -> Bus Creator/1  "Vboost"
  Current Measurement/1 -> Simple Time Delay Sensor 1/1(u)
  Voltage Measurement1/1 -> "Simple Time Delay Sensor "/1(u)
  connections:
  Vpv-/RConn1 -- C1/RConn1 -- Current Measurement/RConn1 -- Mosfet/RConn1
  C1/LConn1 -- Vpv+/RConn1 -- Variable-Ratio Transformer1/LConn1
  Variable-Ratio Transformer1/LConn2 -- Mosfet/LConn1
  Diode2/RConn1 -- Voltage Measurement1/LConn1 -- Vboost+1/RConn1 -- Series RLC Branch3/LConn1
  Variable-Ratio Transformer1/RConn2 -- Current Measurement/LConn1 -- Voltage Measurement1/LConn2 -- Vboost-1/RConn1 -- Series RLC Branch3/RConn1
  Diode2/LConn1 -- Variable-Ratio Transformer1/RConn1

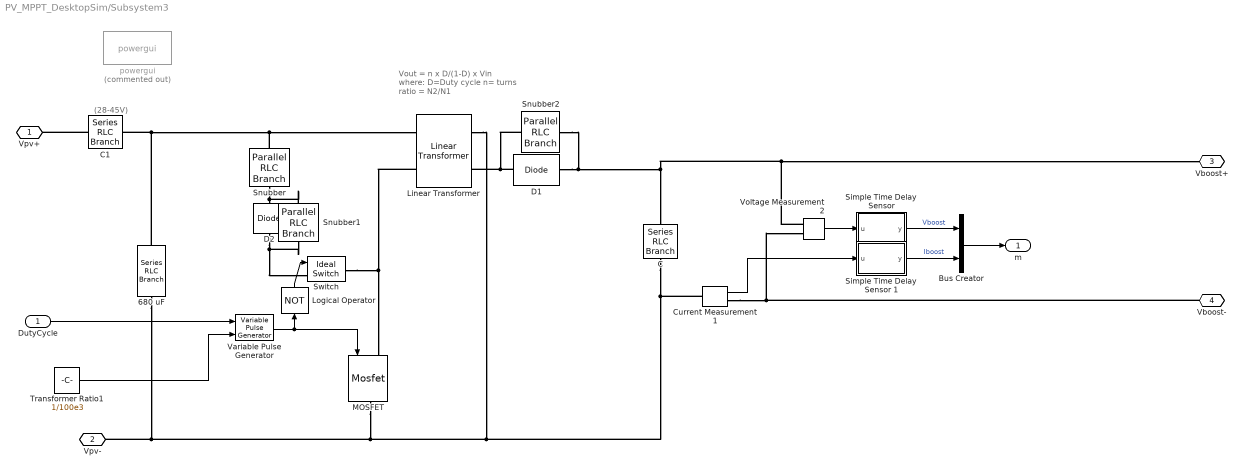
== system PV_MPPT_DesktopSim/Subsystem3 ==
  note: (28-45V)
  note: Vout = n x D/(1-D) x Vin
      | where: D=Duty cycle
      | n= turns ratio = N2/N1
  DutyCycle : Inport
  680 uF : spsSeriesRLCBranchLib/Series RLC Branch  LConnTagsString=__new0  RConnTagsString=__new0  BranchType=C  Resistance=1e-3  Inductance=1e-3  SetiL0=off  InitialCurrent=0  Capacitance=680e-6  Setx0=off  InitialVoltage=20  Measurements=None
  Bus Creator : BusCreator  Inputs=2
  C : spsSeriesRLCBranchLib/Series RLC Branch  LConnTagsString=__new0  RConnTagsString=__new0  BranchType=C  Resistance=1e-4  Inductance=200e-6  SetiL0=off  InitialCurrent=0  Capacitance=1640e-6  Setx0=off  InitialVoltage=0  Measurements=None
  C1 : spsSeriesRLCBranchLib/Series RLC Branch  LConnTagsString=__new0  RConnTagsString=__new0  BranchType=R  Resistance=1e-3  Inductance=200e-6  SetiL0=off  InitialCurrent=0  Capacitance=200e-6  Setx0=off  InitialVoltage=0  Measurements=None
  Current Measurement1 : spsCurrentMeasurementLib/Current Measurement  PhasorSimulation=off  OutputType=Complex  PSBequivalent=0
  D1 : spsDiodeLib/Diode  Ron=1e-3  Lon=0  Vf=0  IC=0  UseSnubber=off  Rs=inf  Cs=0  Measurements=off
  D2 : spsDiodeLib/Diode  Ron=1e-3  Lon=0  Vf=0  IC=0  UseSnubber=off  Rs=inf  Cs=0  Measurements=off
  Linear Transformer : spsLinearTransformerLib/Linear Transformer  UNITS=SI  NominalPower=[50 100e3 ]  winding1=[10 0 0]  winding2=[30 0 0]  ThreeWindings=off  winding3=[3.15e+05 3.969e+07 6316.9]  RmLm=[1e4 1e-3]  Measurements=Magnetization current  DataType=on
  Logical Operator : Logic  Operator=NOT  IconShape=distinctive  AllPortsSameDT=off  OutDataTypeStr=boolean
  MOSFET : spsMosfetLib/Mosfet  Ron=1e-3  Lon=0  Rd=1e-3  Vfd=0  IC=0  Rs=1e6  Cs=inf  Measurements=off
  "Simple Time Delay Sensor " : Subsystem  mask{Ts=Ts, Tau=0.0001}
      mask prompts: Ts "Sample Time, [s]"; Tau "Time Constant, Tau [s]"
      mask help: Simple Sensor
      mask Display: fprintf('1\n------------\n(1 + s Tau)');
  Simple Time Delay Sensor 1 : Subsystem  mask{Ts=Ts, Tau=0.0001}
      mask prompts: Ts "Sample Time, [s]"; Tau "Time Constant, Tau [s]"
      mask help: Simple Sensor
      mask Display: fprintf('1\n------------\n(1 + s Tau)');
  Snubber : spsParallelRLCBranchLib/Parallel RLC Branch  LConnTagsString=a  RConnTagsString=__new0  BranchType=C  Resistance=10e3  Inductance=1e-3  SetiL0=off  InitialCurrent=0  Capacitance=47e-9  Setx0=off  InitialVoltage=0  Measurements=None
  Snubber1 : spsParallelRLCBranchLib/Parallel RLC Branch  LConnTagsString=a  RConnTagsString=__new0  BranchType=R  Resistance=10e6  Inductance=1e-3  SetiL0=off  InitialCurrent=0  Capacitance=47e-9  Setx0=off  InitialVoltage=0  Measurements=None
  Snubber2 : spsParallelRLCBranchLib/Parallel RLC Branch  LConnTagsString=a  RConnTagsString=__new0  BranchType=R  Resistance=10e6  Inductance=1e-3  SetiL0=off  InitialCurrent=0  Capacitance=47e-9  Setx0=off  InitialVoltage=0  Measurements=None
  Switch : spsIdealSwitchLib/Ideal Switch  Ron=0.001  Lon=0  IC=0  Rs=inf  Cs=0  Measurements=off
  Transformer Ratio1 : Constant  Value=1/100e3
  Variable Pulse Generator : VariablePulseGenerator  AllowZeroPulseWidth=on  SampleTime=0.1
  Voltage Measurement2 : spsVoltageMeasurementLib/Voltage Measurement  PhasorSimulation=off  OutputType=Complex  PSBequivalent=0
  powergui : spspowerguiLib/powergui  Priority=1  Commented=on  SimulationMode=Continuous  SampleTime=50e-6  frequency=60  Iterations=50  frequencyindice=0  Pbase=100e6  ErrMax=1e-4  UnitsV=kV  UnitsW=MW  buscounter=0  FunctionMessages=off  echomessages=off  EnableUseOfTLC=off  CurrentSourceSwitches=off  DisableSnubberDevices=off  DisableRonSwitches=off  DisableVfSwitches=off  DisplayEquations=off  AutomaticDiscreteSolvers=off  SolverType=Tustin/Backward Euler (TBE)  Interpol=off  ExternalGateDelay=off  methode=off  Ts=100  x0status=blocks  SPID=on  SwTol=0  HookPort=off  NonlinearTolerance=1e-4  nMaxIteration=100  ContinueOnMaxIteration=off  RestoreLinks=warning  ResistiveCurrentMeasurement=off  Frange=[0:2:500]  Ylog=off  Xlog=on  ShowGrid=off  save=off  variable=ZData  structure=0  ZoomFFT=off  StartTime=0.0  cycles=1  DisplayStyle=1  fundamental=60  FreqAxis=off  MaxFrequency=1000  frequencyindicesteady=1  RmsSteady=1  display=off
  Vpv+ : PMIOPort  Side=Left
  Vpv- : PMIOPort  Port=2  Side=Left
  Vboost+ : PMIOPort  Port=3  Side=Right
  Vboost- : PMIOPort  Port=4  Side=Right
  m : Outport  VectorParamsAs1DForOutWhenUnconnected=off
  wires:
  Variable Pulse Generator/1 -> Logical Operator/1, MOSFET/1
  Simple Time Delay Sensor 1/1(y) -> Bus Creator/2  "Iboost"
  Transformer Ratio1/1 -> Variable Pulse Generator/2
  "Simple Time Delay Sensor "/1(y) -> Bus Creator/1  "Vboost"
  Bus Creator/1 -> m/1
  Voltage Measurement2/1 -> "Simple Time Delay Sensor "/1(u)
  Current Measurement1/1 -> Simple Time Delay Sensor 1/1(u)
  DutyCycle/1 -> Variable Pulse Generator/1
  Logical Operator/1 -> Switch/1
  connections:
  Snubber/RConn1 -- Snubber1/LConn1 -- D2/RConn1
  D1/RConn1 -- C/LConn1 -- Voltage Measurement2/LConn1 -- Vboost+/RConn1 -- Snubber2/LConn1
  Snubber/LConn1 -- Linear Transformer/LConn1 -- 680 uF/LConn1 -- C1/RConn1
  Linear Transformer/RConn1 -- C/RConn1 -- Current Measurement1/LConn1 -- MOSFET/RConn1 -- 680 uF/RConn1 -- Vpv-/RConn1
  Switch/RConn1 -- MOSFET/LConn1 -- Linear Transformer/LConn2
  D1/LConn1 -- Snubber2/RConn1 -- Linear Transformer/RConn2
  D2/LConn1 -- Switch/LConn1 -- Snubber1/RConn1
  C1/LConn1 -- Vpv+/RConn1
  Vboost-/RConn1 -- Current Measurement1/RConn1 -- Voltage Measurement2/LConn2

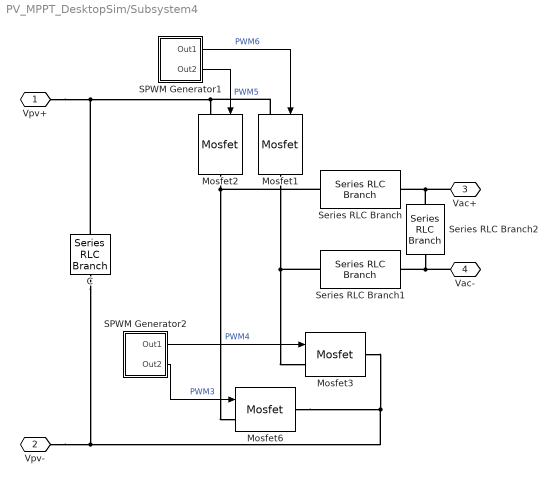
== system PV_MPPT_DesktopSim/Subsystem4 ==
  C : spsSeriesRLCBranchLib/Series RLC Branch  LConnTagsString=__new0  RConnTagsString=__new0  BranchType=C  Resistance=1e-4  Inductance=200e-6  SetiL0=off  InitialCurrent=0  Capacitance=200e-6  Setx0=off  InitialVoltage=0  Measurements=None
  Mosfet{1..3,6} (4 alike) : spsMosfetLib/Mosfet  Ron=0.1  Lon=0  Rd=0.01  Vfd=0  IC=0  Rs=1e5  Cs=inf  Measurements=off
  SPWM Generator1 : Subsystem
  SPWM Generator2 : Subsystem
  Series RLC Branch : spsSeriesRLCBranchLib/Series RLC Branch  LConnTagsString=__new0  RConnTagsString=__new0  BranchType=L  Resistance=1  Inductance=7e-3  SetiL0=off  InitialCurrent=0  Capacitance=1e-6  Setx0=off  InitialVoltage=0  Measurements=None
  Series RLC Branch1 : spsSeriesRLCBranchLib/Series RLC Branch  LConnTagsString=__new0  RConnTagsString=__new0  BranchType=L  Resistance=1  Inductance=7e-3  SetiL0=off  InitialCurrent=0  Capacitance=1e-6  Setx0=off  InitialVoltage=0  Measurements=None
  Series RLC Branch2 : spsSeriesRLCBranchLib/Series RLC Branch  LConnTagsString=__new0  RConnTagsString=__new0  BranchType=C  Resistance=1  Inductance=100e-6  SetiL0=off  InitialCurrent=0  Capacitance=500e-6  Setx0=off  InitialVoltage=0  Measurements=None
  Vpv+ : PMIOPort  Side=Left
  Vpv- : PMIOPort  Port=2  Side=Left
  Vac+ : PMIOPort  Port=3  Side=Right
  Vac- : PMIOPort  Port=4  Side=Right
  wires:
  SPWM Generator2/1(Out1) -> Mosfet3/1  "PWM4"
  SPWM Generator2/2(Out2) -> Mosfet6/1  "PWM3"
  SPWM Generator1/1(Out1) -> Mosfet1/1  "PWM6"
  SPWM Generator1/2(Out2) -> Mosfet2/1  "PWM5"
  connections:
  Mosfet1/RConn1 -- Mosfet3/LConn1 -- Series RLC Branch1/LConn1
  Series RLC Branch2/RConn1 -- Vac-/RConn1 -- Series RLC Branch1/RConn1
  Vpv+/RConn1 -- Mosfet1/LConn1 -- Mosfet2/LConn1 -- C/LConn1
  Series RLC Branch2/LConn1 -- Vac+/RConn1 -- Series RLC Branch/RConn1
  Vpv-/RConn1 -- Mosfet3/RConn1 -- Mosfet6/RConn1 -- C/RConn1
  Mosfet2/RConn1 -- Series RLC Branch/LConn1 -- Mosfet6/LConn1

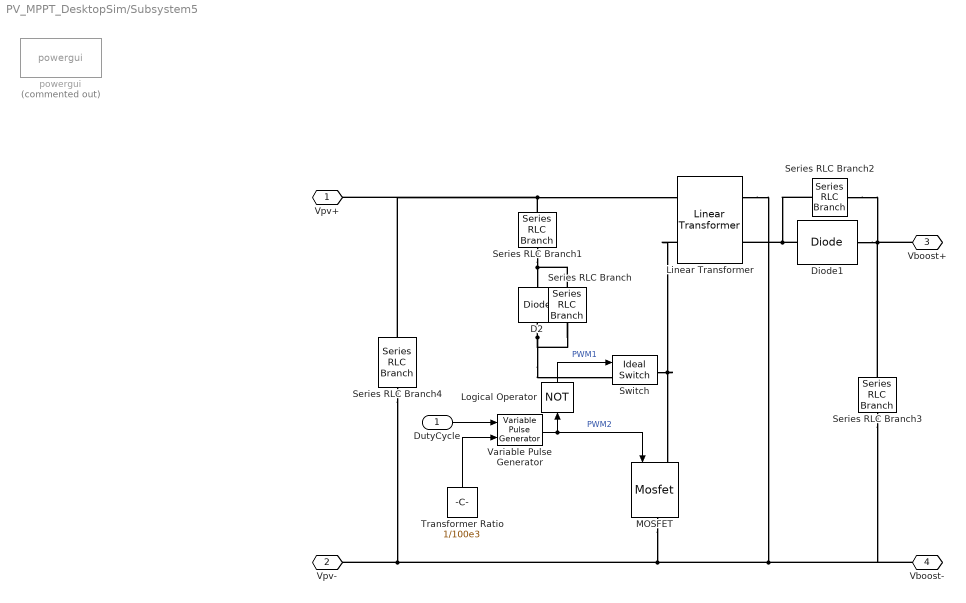
== system PV_MPPT_DesktopSim/Subsystem5 ==
  DutyCycle : Inport
  D2 : spsDiodeLib/Diode  Ron=1e-3  Lon=0  Vf=0  IC=0  UseSnubber=off  Rs=inf  Cs=0  Measurements=off
  Diode1 : spsDiodeLib/Diode  Ron=0.001  Lon=0  Vf=0.8  IC=0  UseSnubber=0  Rs=inf  Cs=250e-9  Measurements=off
  Linear Transformer : spsLinearTransformerLib/Linear Transformer  UNITS=SI  NominalPower=[50 100e3 ]  winding1=[10 0 0]  winding2=[30 0 0]  ThreeWindings=off  winding3=[3.15e+05 3.969e+07 6316.9]  RmLm=[1e4 1e-3]  Measurements=Magnetization current  DataType=on
  Logical Operator : Logic  Operator=NOT  IconShape=distinctive  AllPortsSameDT=off  OutDataTypeStr=boolean
  MOSFET : spsMosfetLib/Mosfet  Ron=1e-3  Lon=0  Rd=1e-3  Vfd=0  IC=0  Rs=1e6  Cs=inf  Measurements=off
  Series RLC Branch : spsSeriesRLCBranchLib/Series RLC Branch  LConnTagsString=__new0  RConnTagsString=__new0  BranchType=R  Resistance=1  Inductance=1e-3  SetiL0=off  InitialCurrent=0  Capacitance=1e-6  Setx0=off  InitialVoltage=0  Measurements=None
  Series RLC Branch1 : spsSeriesRLCBranchLib/Series RLC Branch  LConnTagsString=__new0  RConnTagsString=__new0  BranchType=C  Resistance=1  Inductance=1e-3  SetiL0=off  InitialCurrent=0  Capacitance=1e-6  Setx0=off  InitialVoltage=0  Measurements=None
  Series RLC Branch2 : spsSeriesRLCBranchLib/Series RLC Branch  LConnTagsString=__new0  RConnTagsString=__new0  BranchType=R  Resistance=1  Inductance=1e-3  SetiL0=off  InitialCurrent=0  Capacitance=1e-6  Setx0=off  InitialVoltage=0  Measurements=None
  Series RLC Branch3 : spsSeriesRLCBranchLib/Series RLC Branch  LConnTagsString=__new0  RConnTagsString=__new0  BranchType=C  Resistance=1  Inductance=1e-3  SetiL0=off  InitialCurrent=0  Capacitance=1e-6  Setx0=off  InitialVoltage=0  Measurements=None
  Series RLC Branch4 : spsSeriesRLCBranchLib/Series RLC Branch  LConnTagsString=__new0  RConnTagsString=__new0  BranchType=C  Resistance=1  Inductance=1e-3  SetiL0=off  InitialCurrent=0  Capacitance=1e-6  Setx0=off  InitialVoltage=0  Measurements=None
  Switch : spsIdealSwitchLib/Ideal Switch  Ron=0.001  Lon=0  IC=0  Rs=inf  Cs=0  Measurements=off
  Transformer Ratio : Constant  Value=1/100e3
  Variable Pulse Generator : VariablePulseGenerator  AllowZeroPulseWidth=on  SampleTime=0.1
  powergui : spspowerguiLib/powergui  Priority=1  Commented=on  SimulationMode=Continuous  SampleTime=50e-6  frequency=60  Iterations=50  frequencyindice=0  Pbase=100e6  ErrMax=1e-4  UnitsV=kV  UnitsW=MW  buscounter=0  FunctionMessages=off  echomessages=off  EnableUseOfTLC=off  CurrentSourceSwitches=off  DisableSnubberDevices=off  DisableRonSwitches=off  DisableVfSwitches=off  DisplayEquations=off  AutomaticDiscreteSolvers=off  SolverType=Tustin/Backward Euler (TBE)  Interpol=off  ExternalGateDelay=off  methode=off  Ts=100  x0status=blocks  SPID=on  SwTol=0  HookPort=off  NonlinearTolerance=1e-4  nMaxIteration=100  ContinueOnMaxIteration=off  RestoreLinks=warning  ResistiveCurrentMeasurement=off  Frange=[0:2:500]  Ylog=off  Xlog=on  ShowGrid=off  save=off  variable=ZData  structure=0  ZoomFFT=off  StartTime=0.0  cycles=1  DisplayStyle=1  fundamental=60  FreqAxis=off  MaxFrequency=1000  frequencyindicesteady=1  RmsSteady=1  display=off
  Vpv+ : PMIOPort  Side=Left
  Vpv- : PMIOPort  Port=2  Side=Left
  Vboost+ : PMIOPort  Port=3  Side=Right
  Vboost- : PMIOPort  Port=4  Side=Right
  wires:
  Variable Pulse Generator/1 -> MOSFET/1, Logical Operator/1  "PWM2"
  Transformer Ratio/1 -> Variable Pulse Generator/2
  DutyCycle/1 -> Variable Pulse Generator/1
  Logical Operator/1 -> Switch/1  "PWM1"
  connections:
  Series RLC Branch/LConn1 -- Series RLC Branch1/RConn1 -- D2/RConn1
  Vboost+/RConn1 -- Series RLC Branch2/LConn1 -- Series RLC Branch3/LConn1 -- Diode1/RConn1
  Linear Transformer/RConn1 -- Vboost-/RConn1 -- Series RLC Branch3/RConn1 -- MOSFET/RConn1 -- Series RLC Branch4/RConn1 -- Vpv-/RConn1
  Linear Transformer/LConn2 -- Switch/RConn1 -- MOSFET/LConn1
  Series RLC Branch2/RConn1 -- Linear Transformer/RConn2 -- Diode1/LConn1
  D2/LConn1 -- Series RLC Branch/RConn1 -- Switch/LConn1
  Series RLC Branch4/LConn1 -- Vpv+/RConn1 -- Series RLC Branch1/LConn1 -- Linear Transformer/LConn1

== system PV_MPPT_DesktopSim/Boost Converter/Simple Time Delay Sensor  ==
  u : Inport
  1/Tau : Gain  Gain=1/Tau
  Discrete-Time Integrator : DiscreteIntegrator  SampleTime=Ts  ICPrevOutput=DiscIntNeverNeededParam  ICPrevScaledInput=DiscIntNeverNeededParam
  Sum : Sum  Inputs=|+-
  y : Outport  VectorParamsAs1DForOutWhenUnconnected=off
  wires:
  Discrete-Time Integrator/1 -> Sum/2, y/1
  u/1 -> Sum/1
  Sum/1 -> 1/Tau/1
  1/Tau/1 -> Discrete-Time Integrator/1

== system PV_MPPT_DesktopSim/Boost Converter/Simple Time Delay Sensor 1 ==
  u : Inport
  1/Tau : Gain  Gain=1/Tau
  Discrete-Time Integrator : DiscreteIntegrator  SampleTime=Ts  ICPrevOutput=DiscIntNeverNeededParam  ICPrevScaledInput=DiscIntNeverNeededParam
  Sum : Sum  Inputs=|+-
  y : Outport  VectorParamsAs1DForOutWhenUnconnected=off
  wires:
  1/Tau/1 -> Discrete-Time Integrator/1
  Sum/1 -> 1/Tau/1
  u/1 -> Sum/1
  Discrete-Time Integrator/1 -> y/1, Sum/2

== system PV_MPPT_DesktopSim/Emulated PV Panel Lookup Table/Ifilter ==
  u : Inport
  1/T6 : Gain  Gain=1/Tf
  Discrete-Time Integrator : DiscreteIntegrator  SampleTime=Tc  ICPrevOutput=DiscIntNeverNeededParam  ICPrevScaledInput=DiscIntNeverNeededParam
  Sum1 : Sum  Inputs=|+-
  y : Outport  VectorParamsAs1DForOutWhenUnconnected=off
  wires:
  Sum1/1 -> 1/T6/1
  Discrete-Time Integrator/1 -> Sum1/2, y/1
  u/1 -> Sum1/1
  1/T6/1 -> Discrete-Time Integrator/1

== system PV_MPPT_DesktopSim/Emulated PV Panel Lookup Table/Simple Time Delay Sensor ==
  u : Inport
  1/Tau : Gain  Gain=1/Tau
  Discrete-Time Integrator : DiscreteIntegrator  SampleTime=Ts  ICPrevOutput=DiscIntNeverNeededParam  ICPrevScaledInput=DiscIntNeverNeededParam
  Sum : Sum  Inputs=|+-
  y : Outport  VectorParamsAs1DForOutWhenUnconnected=off
  wires:
  1/Tau/1 -> Discrete-Time Integrator/1
  Sum/1 -> 1/Tau/1
  u/1 -> Sum/1
  Discrete-Time Integrator/1 -> y/1, Sum/2

== system PV_MPPT_DesktopSim/Emulated PV Panel Lookup Table/Simple Time Delay Sensor  ==
  u : Inport
  1/Tau : Gain  Gain=1/Tau
  Discrete-Time Integrator : DiscreteIntegrator  SampleTime=Ts  ICPrevOutput=DiscIntNeverNeededParam  ICPrevScaledInput=DiscIntNeverNeededParam
  Sum : Sum  Inputs=|+-
  y : Outport  VectorParamsAs1DForOutWhenUnconnected=off
  wires:
  Discrete-Time Integrator/1 -> Sum/2, y/1
  u/1 -> Sum/1
  Sum/1 -> 1/Tau/1
  1/Tau/1 -> Discrete-Time Integrator/1

== system PV_MPPT_DesktopSim/Emulated PV Panel Lookup Table/Vfilter ==
  u : Inport
  1/T6 : Gain  Gain=1/Tf
  Discrete-Time Integrator : DiscreteIntegrator  SampleTime=Tc  ICPrevOutput=DiscIntNeverNeededParam  ICPrevScaledInput=DiscIntNeverNeededParam
  Sum1 : Sum  Inputs=|+-
  y : Outport  VectorParamsAs1DForOutWhenUnconnected=off
  wires:
  1/T6/1 -> Discrete-Time Integrator/1
  u/1 -> Sum1/1
  Discrete-Time Integrator/1 -> y/1, Sum1/2
  Sum1/1 -> 1/T6/1

== system PV_MPPT_DesktopSim/MPPT and Boost Controllers/Digital Pulse ==
  Freq : Inport
  Compare To Constant : simulink/Logic and Bit Operations/Compare To Constant  relop=>=  const=Duty  OutDataTypeStr=boolean
  Constant1 : Constant
  Discrete-Time Integrator : DiscreteIntegrator  ExternalReset=rising  SampleTime=Ts  ShowStatePort=on  ICPrevOutput=DiscIntNeverNeededParam  ICPrevScaledInput=DiscIntNeverNeededParam
  Relational Operator1 : RelationalOperator  Operator=>  OutDataTypeStr=boolean  InputSameDT=off
  Pulse : Outport  VectorParamsAs1DForOutWhenUnconnected=off
  wires:
  Relational Operator1/1 -> Discrete-Time Integrator/2
  Constant1/1 -> Relational Operator1/2
  Compare To Constant/1 -> Pulse/1
  Discrete-Time Integrator/State -> Relational Operator1/1
  Discrete-Time Integrator/1 -> Compare To Constant/1
  Freq/1 -> Discrete-Time Integrator/1
